simulink library "common_lib"  (R2021b)
settings: Solver=ode45  StartTime=0.0  StopTime=10.0  RelTol=1e-3
undefined symbols (not defined in the file or in its folder): ACCEL_PRE_MULT, C_C1GearNumbers, C_C1GearRatios, C_Calibration, C_DitherWaveform, C_GearOffset, C_GearRatioIn, C_GearRatioInverseOut, C_GearRatioOut, CLUTCH_INNER_LOOP_UPDATE_RATE, CONSTANT, DEGRADED_MODE_SIZE, Dem_EventStatusType, DiscIntNeverNeededParam, F_FAULT_ENUM, F_NOFAULT, F_OUTOFRANGE, F_RATELIMIT, FALSE, FMI14_SPECIAL_INSTRUCTIONS, FMI20_DATA_DRIFTED_HIGH, FMI21_DATA_DRIFTED_LOW, FMI29_RESERVED_FOR_SAE_ASSIGNMENT, FMI30_RESERVED_FOR_SAE_ASSIGNMENT, FMI31_CONDITION_EXISTS, FMI32_NO_FAULT, IC, k_accel, k_mean, LVDCU_OORH_FaultCntThd_C, MAX_UINT32, MEAN_PRE_MULT, NTriggers, QLTY_SIGNAL_FAILED, QLTY_SIGNAL_FULLY_FUNCTION, QLTY_SIGNAL_SUBSTITUTED_BY_1ST_CHOICE, QLTY_SIGNAL_SUBSTITUTED_BY_2ND_CHOICE, QLTY_SIGNAL_SUBSTITUTED_BY_3RD_CHOICE, QLTY_SIGNAL_SUBSTITUTED_BY_4TH_CHOICE, SAMPLE_TIME_100_mSec, SAMPLE_TIME_100_uSec, simin, T_TestPoint, TF_FALSE, TF_TRUE, TimeStep, TRUE, WORKSPACE_UPDATE_RATE, ZERO, Zero
libraries: $bdroot x120, simulink x27, simulink_extras x4, MBD_EPS_Local_Blockset x4
(part 5 of 10)

== system common_lib/Diagnostics/Calibration Enabled Debounce ==
  diagInput : Inport
  diagStartUpComp : Inport  Port=2
  diagMaxVal : Inport  Port=3
  diagMinVal : Inport  Port=4
  diagUpCnt : Inport  Port=5
  diagDnCnt : Inport  Port=6
  diagFaultCntThresh : Inport  Port=7
  diagPassCntThresh : Inport  Port=8
  diagDbncEnab : Inport  Port=9
  diagReset : Inport  Port=10
  diagEnable : Inport  Port=11
  diagHealEn : Inport  Port=12
  Calibration Enabled Debounce Boolean Input : $bdroot/Diagnostics/Calibration Enabled Debounce Boolean Input  SystemSampleTime=-1  VariantActivationTime=update diagram  Latency=0  AutoFrameSizeCalculation=off
  OR : Logic  Operator=OR  AllPortsSameDT=off  OutDataTypeStr=boolean
  Relational Operator : RelationalOperator  OutDataTypeStr=boolean  ZeroCross=off  RndMeth=Nearest
  Relational Operator1 : RelationalOperator  Operator=<=  OutDataTypeStr=boolean  ZeroCross=off  RndMeth=Nearest
  diagFaultStatus : Outport  OutputWhenDisabled=reset  InitialOutput=Dem_EventStatusType.DEM_EVENT_STATUS_INIT  VectorParamsAs1DForOutWhenUnconnected=off
  wires:
  diagHealEn/1 -> Calibration Enabled Debounce Boolean Input/10
  diagPassCntThresh/1 -> Calibration Enabled Debounce Boolean Input/7
  diagMaxVal/1 -> Relational Operator/2
  diagMinVal/1 -> Relational Operator1/2
  Relational Operator/1 -> OR/1
  Relational Operator1/1 -> OR/2
  diagInput/1 -> Relational Operator/1, Relational Operator1/1
  OR/1 -> Calibration Enabled Debounce Boolean Input/1
  diagStartUpComp/1 -> Calibration Enabled Debounce Boolean Input/2
  diagReset/1 -> Calibration Enabled Debounce Boolean Input/3
  diagEnable/1 -> Calibration Enabled Debounce Boolean Input/4
  diagDbncEnab/1 -> Calibration Enabled Debounce Boolean Input/5
  diagFaultCntThresh/1 -> Calibration Enabled Debounce Boolean Input/6
  diagUpCnt/1 -> Calibration Enabled Debounce Boolean Input/8
  diagDnCnt/1 -> Calibration Enabled Debounce Boolean Input/9
  Calibration Enabled Debounce Boolean Input/1 -> diagFaultStatus/1

== system common_lib/Diagnostics/Calibration Enabled Debounce Boolean Input ==
  diagInput : Inport
  diagStartUpComp : Inport  Port=2
  diagUpCnt : Inport  Port=3
  diagDnCnt : Inport  Port=4
  diagFaultCntThresh : Inport  Port=5
  diagPassCntThresh : Inport  Port=6
  diagDbncEnab : Inport  Port=7
  diagReset : Inport  Port=8
  diagEnable : Inport  Port=9
  diagHealEn : Inport  Port=10
  DiagFaultCounter : Subsystem
  diagFaultStatus : Outport  OutputWhenDisabled=reset  InitialOutput=Dem_EventStatusType.DEM_EVENT_STATUS_INIT  VectorParamsAs1DForOutWhenUnconnected=off
  diagFaultCnt : Outport  Port=2  OutputWhenDisabled=reset  InitialOutput=Dem_EventStatusType.DEM_EVENT_STATUS_INIT  VectorParamsAs1DForOutWhenUnconnected=off
  wires:
  DiagFaultCounter/1(diagFaultStatus) -> diagFaultStatus/1
  diagDnCnt/1 -> DiagFaultCounter/9(diagDnCnt)
  diagUpCnt/1 -> DiagFaultCounter/8(diagUpCnt)
  diagFaultCntThresh/1 -> DiagFaultCounter/6(diagFaultCntThresh)
  diagDbncEnab/1 -> DiagFaultCounter/5(diagDbncEnab)
  diagEnable/1 -> DiagFaultCounter/4(diagEnable)
  diagReset/1 -> DiagFaultCounter/3(diagReset)
  diagStartUpComp/1 -> DiagFaultCounter/2(diagStartUpComp)
  diagInput/1 -> DiagFaultCounter/1(diagFaultActive)
  diagPassCntThresh/1 -> DiagFaultCounter/7(diagPassCntThresh)
  diagHealEn/1 -> DiagFaultCounter/10(diagHealEn)
  DiagFaultCounter/2(diagFaultCnt) -> diagFaultCnt/1

== system common_lib/Diagnostics/Calibration Enabled MinMax OOR ==
  Input : Inport
  ULim : Inport  Port=2
  LLim : Inport  Port=3
  Cal_Enable : Inport  Port=4
  Ext_Fault : Inport  Port=5
  Enabled OOR : Subsystem  mask(Enabled OOR Subsystem){InitialValue=InitialValue, InDataType=single}
      mask prompts: InitialValue "Initial Value"; InDataType "Input Data Type"
      mask init:
      | DataType = get_param(gcb, 'InDataType');
      | Capture1 = [gcb '/OOR MinMax Capture/CL MinMax Capture'];
      | Capture2 = [gcb '/OOR MinMax Capture/CL MinMax Capture1'];
      | 
      | set_param(Capture1, 'InDataType', DataType);
      | set_param(Capture2, 'InDataType', DataType);
      mask TypeOptions InDataType: single | int16
  Switch : Switch  Threshold=0.5  ZeroCross=off
  Switch1 : Switch  Threshold=0.5  ZeroCross=off
  Out : Outport  VectorParamsAs1DForOutWhenUnconnected=off
  Max_Value : Outport  Port=2  VectorParamsAs1DForOutWhenUnconnected=off
  Min_Value : Outport  Port=3  VectorParamsAs1DForOutWhenUnconnected=off
  Fault : Outport  Port=4  VectorParamsAs1DForOutWhenUnconnected=off
  wires:
  Input/1 -> Enabled OOR/1(In), Switch/3
  ULim/1 -> Enabled OOR/2(ULim)
  LLim/1 -> Enabled OOR/3(LLim)
  Ext_Fault/1 -> Enabled OOR/4(Ext_Fault), Switch1/3
  Switch/1 -> Out/1
  Switch1/1 -> Fault/1
  Enabled OOR/1(Out) -> Switch/1
  Cal_Enable/1 -> Switch1/2, Switch/2, Enabled OOR/Enable
  Enabled OOR/2(Fault) -> Switch1/1
  Enabled OOR/3(Max) -> Max_Value/1
  Enabled OOR/4(Min) -> Min_Value/1

== system common_lib/Diagnostics/Calibration Enabled MinMax RLim ==
  Input : Inport
  Rate_Limit : Inport  Port=2
  Cal_Enable : Inport  Port=3
  Ext_Fault : Inport  Port=4
  Enabled RLim : Subsystem  mask(Enablede Rate Limit Fault Detection){IC=IC, TimeStep=TimeStep, InDataType=single}
      mask prompts: IC "Initial Condition"; TimeStep "Update Time"; InDataType "Input Data Type"
      mask init:
      | DataType = get_param(gcb, 'InDataType');
      | Capture1 = [gcb '/RLim MinMax Capture/CL MinMax Capture'];
      | Capture2 = [gcb '/RLim MinMax Capture/CL MinMax Capture1'];
      | 
      | set_param(Capture1, 'InDataType', DataType);
      | set_param(Capture2, 'InDataType', DataType);
      mask TypeOptions InDataType: single | int16
  Switch : Switch  Threshold=0.5  ZeroCross=off
  Switch1 : Switch  Threshold=0.5  ZeroCross=off
  Out : Outport  VectorParamsAs1DForOutWhenUnconnected=off
  Max Pos Rate : Outport  Port=2  VectorParamsAs1DForOutWhenUnconnected=off
  Max Neg Rate : Outport  Port=3  VectorParamsAs1DForOutWhenUnconnected=off
  Fault : Outport  Port=4  VectorParamsAs1DForOutWhenUnconnected=off
  wires:
  Cal_Enable/1 -> Switch/2, Switch1/2, Enabled RLim/Enable
  Input/1 -> Switch/3, Enabled RLim/1(In)
  Switch/1 -> Out/1
  Switch1/1 -> Fault/1
  Rate_Limit/1 -> Enabled RLim/2(RLim)
  Enabled RLim/1(out) -> Switch/1
  Enabled RLim/2(fault?) -> Switch1/1
  Ext_Fault/1 -> Enabled RLim/3(Ext_Fault), Switch1/3
  Enabled RLim/3(Max Pos Rate) -> Max Pos Rate/1
  Enabled RLim/4(Max Neg Rate) -> Max Neg Rate/1

== system common_lib/Diagnostics/Ccaller_DiagLv1 ==
  diagFaultActive : Inport
  diagStartUpComp : Inport  Port=2
  diagReset : Inport  Port=3
  diagEnable : Inport  Port=4
  diagDbncEnable : Inport  Port=5
  diagFaultCntThresh : Inport  Port=6
  diagPassCntThresh : Inport  Port=7
  diagUpCnt : Inport  Port=8
  diagDnCnt : Inport  Port=9
  diagHealEn : Inport  Port=10
  DiagDebounceLv1_CCaller : CCaller  FunctionName=DiagDebounceLv1  PortSpecificationStruct="%)30     .    <!<   8    (     @         %    \"     T    !     0         %  0 \"0    $    _    07)G3F%M90  4&]R=$YA;64 4V-O<&4     26YD97@     5'EP90      4VEZ90      27-';&]B86P   X   !     !@    @    $          4    (     0   !     !         !     0    9&EA9T9A=6QT0V]U;G1E<@X   !     !@    @    $          4    (     0   !     !         !     0    9&EA9T9A=6QT0V]U;G1E<@X   !     !@    @    $     ...(+7711 chars)"
  Unit Delay : UnitDelay  SampleTime=-1  HasFrameUpgradeWarning=on
      settings: AttributesFormatString=%<InitialCondition>
  Unit Delay1 : UnitDelay  InitialCondition=uint8(32)  SampleTime=-1  HasFrameUpgradeWarning=on
      settings: AttributesFormatString=%<InitialCondition>
  Unit Delay2 : UnitDelay  InitialCondition=false  SampleTime=-1  HasFrameUpgradeWarning=on
      settings: AttributesFormatString=%<InitialCondition>
  diagFaultStatus : Outport  VectorParamsAs1DForOutWhenUnconnected=off
  wires:
  diagUpCnt/1 -> DiagDebounceLv1_CCaller/11
  diagStartUpComp/1 -> DiagDebounceLv1_CCaller/5
  diagDnCnt/1 -> DiagDebounceLv1_CCaller/12
  diagReset/1 -> DiagDebounceLv1_CCaller/6
  diagFaultCntThresh/1 -> DiagDebounceLv1_CCaller/9
  diagFaultActive/1 -> DiagDebounceLv1_CCaller/4
  diagHealEn/1 -> DiagDebounceLv1_CCaller/13
  diagEnable/1 -> DiagDebounceLv1_CCaller/7
  diagDbncEnable/1 -> DiagDebounceLv1_CCaller/8
  diagPassCntThresh/1 -> DiagDebounceLv1_CCaller/10
  DiagDebounceLv1_CCaller/2 -> diagFaultStatus/1, Unit Delay1/1
  Unit Delay/1 -> DiagDebounceLv1_CCaller/1
  Unit Delay1/1 -> DiagDebounceLv1_CCaller/2
  DiagDebounceLv1_CCaller/3 -> Unit Delay2/1
  Unit Delay2/1 -> DiagDebounceLv1_CCaller/3
  DiagDebounceLv1_CCaller/1 -> Unit Delay/1

== system common_lib/Diagnostics/Ccaller_DiagLv2 ==
  diagFaultActive : Inport
  diagStartUpComp : Inport  Port=2
  diagReset : Inport  Port=3
  diagFaultCntThresh : Inport  Port=4
  diagUpCnt : Inport  Port=5
  diagDnCnt : Inport  Port=6
  diagHealEn : Inport  Port=7
  DiagDebounceLv2_CCaller : CCaller  FunctionName=DiagDebounceLv2  PortSpecificationStruct="%)30     .    8!$   8    (     @         %    \"     L    !     0         %  0 \"0    $    V    07)G3F%M90  4&]R=$YA;64 4V-O<&4     26YD97@     5'EP90      4VEZ90         .    ,     8    (    !          %    \"     $    #     0         0  , ;W5T  X    P    !@    @    $          4    (     0    ,    !         !   P!O=70 #@   #@    &    \"     0         !0    @    !    !@    $         $     8   !/=7 ...(+5614 chars)"
  Unit Delay : UnitDelay  InitialCondition=int16(0)  SampleTime=-1  HasFrameUpgradeWarning=on
      settings: AttributesFormatString=%<InitialCondition>
  Unit Delay1 : UnitDelay  InitialCondition=uint8(0)  SampleTime=-1  HasFrameUpgradeWarning=on
      settings: AttributesFormatString=%<InitialCondition>
  Unit Delay2 : UnitDelay  InitialCondition=int16(0)  SampleTime=-1  HasFrameUpgradeWarning=on
      settings: AttributesFormatString=%<InitialCondition>
  diagFaultStatus : Outport  VectorParamsAs1DForOutWhenUnconnected=off
  wires:
  Unit Delay2/1 -> DiagDebounceLv2_CCaller/3
  DiagDebounceLv2_CCaller/4 -> Unit Delay2/1
  Unit Delay1/1 -> DiagDebounceLv2_CCaller/2
  DiagDebounceLv2_CCaller/3 -> Unit Delay1/1
  Unit Delay/1 -> DiagDebounceLv2_CCaller/1
  DiagDebounceLv2_CCaller/2 -> Unit Delay/1
  diagHealEn/1 -> DiagDebounceLv2_CCaller/10
  diagFaultActive/1 -> DiagDebounceLv2_CCaller/4
  diagFaultCntThresh/1 -> DiagDebounceLv2_CCaller/7
  DiagDebounceLv2_CCaller/1 -> diagFaultStatus/1
  diagReset/1 -> DiagDebounceLv2_CCaller/6
  diagDnCnt/1 -> DiagDebounceLv2_CCaller/9
  diagStartUpComp/1 -> DiagDebounceLv2_CCaller/5
  diagUpCnt/1 -> DiagDebounceLv2_CCaller/8

== system common_lib/Diagnostics/DTNA_Diag ==
  diagInput : Inport
  diagStartUpComp : Inport  Port=2
  diagUpCnt : Inport  Port=3
  diagDnCnt : Inport  Port=4
  diagFaultCntThresh : Inport  Port=5
  diagPassCntThresh : Inport  Port=6
  diagDbncEnab : Inport  Port=7
  diagReset : Inport  Port=8
  diagEnable : Inport  Port=9
  diagHealEn : Inport  Port=10
  CC_Diag : Subsystem  VariantControl=CC_Diag
  S_Diag : Subsystem  AncestorBlock=common_lib/Diagnostics/Calibration Enabled Debounce Boolean Input  VariantControl=S_Diag
      settings: RTWSystemCode=Inline
  diagFaultStatus : Outport
  diagFaultCnt : Outport  Port=2

== system common_lib/Diagnostics/DiagFaultCounter ==
  diagFaultActive : Inport
  diagStartUpComp : Inport  Port=2
  diagReset : Inport  Port=3
  diagEnable : Inport  Port=4
  diagDbncEnab : Inport  Port=5
  diagFaultCntThresh : Inport  Port=6
  diagPassCntThresh : Inport  Port=7
  diagUpCnt : Inport  Port=8
  diagDnCnt : Inport  Port=9
  diagHealEn : Inport  Port=10
  DiagFaulCounter : Stateflow chart  TreatAsAtomicUnit=on
  diagFaultStatus : Outport  OutputWhenDisabled=reset  InitialOutput=Dem_EventStatusType.DEM_EVENT_STATUS_INIT  VectorParamsAs1DForOutWhenUnconnected=off
  wires:
  diagHealEn/1 -> DiagFaulCounter/10(diagHealEn)
  diagPassCntThresh/1 -> DiagFaulCounter/7(diagPassCntThresh)
  diagStartUpComp/1 -> DiagFaulCounter/2(diagStartUpComp)
  diagDbncEnab/1 -> DiagFaulCounter/5(diagDbncEnab)
  DiagFaulCounter/1(diagFaultStatus) -> diagFaultStatus/1
  diagEnable/1 -> DiagFaulCounter/4(diagEnable)
  diagDnCnt/1 -> DiagFaulCounter/9(diagDnCnt)
  diagUpCnt/1 -> DiagFaulCounter/8(diagUpCnt)
  diagReset/1 -> DiagFaulCounter/3(diagReset)
  diagFaultCntThresh/1 -> DiagFaulCounter/6(diagFaultCntThresh)
  diagFaultActive/1 -> DiagFaulCounter/1(diagFaultActive)

== system common_lib/Diagnostics/DiagcFltCumCnt ==
  diaginput : Inport
  diagStartUpComp : Inport  Port=2
  diagFaultCntThresh : Inport  Port=3
  diagReset : Inport  Port=4
  Add2 : Sum
  Constant{3,5,10..11} (4 alike) : Constant  Value=0
  Constant9 : Constant
  GreaterThanOrEqual2 : RelationalOperator  OutDataTypeStr=boolean  RndMeth=Simplest
  GreaterThanOrEqual3 : RelationalOperator  OutDataTypeStr=boolean  RndMeth=Simplest
  Increment Stored Integer1 : simulink/Additional Math & Discrete/Additional Math: Increment - Decrement/Increment Stored Integer
  Switch10 : Switch  Criteria=u2 ~= 0  Threshold=LVDCU_OORH_FaultCntThd_C  OutDataTypeStr=Inherit: Inherit via back propagation
  Switch11 : Switch  Criteria=u2 ~= 0  Threshold=LVDCU_OORH_FaultCntThd_C  OutDataTypeStr=Inherit: Inherit via back propagation
  Switch7 : Switch  Criteria=u2 ~= 0  Threshold=LVDCU_OORH_FaultCntThd_C +1
  Switch8 : Switch  Criteria=u2 > Threshold
  Switch9 : Switch  Criteria=u2 ~= 0  Threshold=1
  Unit Delay1 : UnitDelay  SampleTime=-1  HasFrameUpgradeWarning=on
  Unit Delay4 : UnitDelay  SampleTime=-1  HasFrameUpgradeWarning=on
  diagfaultStatus : Outport
  wires:
  Switch8/1 -> Switch9/3
  diaginput/1 -> Switch8/1
  diagStartUpComp/1 -> Switch8/3, Switch8/2
  Increment Stored Integer1/1 -> GreaterThanOrEqual2/2
  GreaterThanOrEqual2/1 -> Switch7/2
  Constant3/1 -> Switch7/1
  Constant5/1 -> Switch9/1
  Switch9/1 -> Add2/1
  Add2/1 -> GreaterThanOrEqual2/1, Switch7/3
  Unit Delay1/1 -> Add2/2
  Switch7/1 -> GreaterThanOrEqual3/1, Unit Delay1/1  "fault_count"
  diagFaultCntThresh/1 -> Increment Stored Integer1/1, GreaterThanOrEqual3/2
  GreaterThanOrEqual3/1 -> Switch10/2
  Constant9/1 -> Switch10/1
  Constant10/1 -> Switch10/3
  Switch11/1 -> Unit Delay4/1, diagfaultStatus/1
  diagReset/1 -> Switch11/2
  Switch10/1 -> Switch11/3
  Constant11/1 -> Switch11/1
  Unit Delay4/1 -> Switch9/2

== system common_lib/Diagnostics/DiagcFltCumUpCnt ==
  diaginput : Inport
  diagStartUpComp : Inport  Port=2
  diagUpCnt : Inport  Port=3
  diagFaultCntThresh : Inport  Port=4
  diagReset : Inport  Port=5
  Add2 : Sum
  Constant{3,5,10..11} (4 alike) : Constant  Value=0
  Constant9 : Constant
  Equal : RelationalOperator  Operator===  OutDataTypeStr=boolean  RndMeth=Simplest
  GreaterThanOrEqual2 : RelationalOperator  OutDataTypeStr=boolean  RndMeth=Simplest
  GreaterThanOrEqual3 : RelationalOperator  OutDataTypeStr=boolean  RndMeth=Simplest
  Increment Stored Integer1 : simulink/Additional Math & Discrete/Additional Math: Increment - Decrement/Increment Stored Integer
  Switch10 : Switch  Criteria=u2 ~= 0  Threshold=LVDCU_OORH_FaultCntThd_C  OutDataTypeStr=Inherit: Inherit via back propagation
  Switch11 : Switch  Criteria=u2 ~= 0  Threshold=LVDCU_OORH_FaultCntThd_C  OutDataTypeStr=Inherit: Inherit via back propagation
  Switch7 : Switch  Criteria=u2 ~= 0  Threshold=LVDCU_OORH_FaultCntThd_C +1
  Switch8 : Switch  Criteria=u2 > Threshold
  Switch9 : Switch  Criteria=u2 ~= 0  Threshold=1
  Unit Delay1 : UnitDelay  SampleTime=-1  HasFrameUpgradeWarning=on
  Unit Delay4 : UnitDelay  SampleTime=-1  HasFrameUpgradeWarning=on
  diagfaultStatus : Outport
  diagfaultCnt : Outport  Port=2
  wires:
  diagUpCnt/1 -> Equal/2
  Equal/1 -> Switch9/3
  Switch8/1 -> Equal/1
  diaginput/1 -> Switch8/1
  diagStartUpComp/1 -> Switch8/3, Switch8/2
  Increment Stored Integer1/1 -> GreaterThanOrEqual2/2
  GreaterThanOrEqual2/1 -> Switch7/2
  Constant3/1 -> Switch7/1
  Constant5/1 -> Switch9/1
  Switch9/1 -> Add2/1
  Add2/1 -> GreaterThanOrEqual2/1, Switch7/3
  Unit Delay1/1 -> Add2/2
  Switch7/1 -> diagfaultCnt/1, GreaterThanOrEqual3/1, Unit Delay1/1  "fault_count"
  diagFaultCntThresh/1 -> Increment Stored Integer1/1, GreaterThanOrEqual3/2
  GreaterThanOrEqual3/1 -> Switch10/2
  Constant9/1 -> Switch10/1
  Constant10/1 -> Switch10/3
  Switch11/1 -> Unit Delay4/1, diagfaultStatus/1
  diagReset/1 -> Switch11/2
  Switch10/1 -> Switch11/3
  Constant11/1 -> Switch11/1
  Unit Delay4/1 -> Switch9/2

== system common_lib/Diagnostics/DiagcFltResetCnt ==
  diaginput : Inport
  diagStartUpComp : Inport  Port=2
  diagFaultCntThresh : Inport  Port=3
  diagReset : Inport  Port=4
  Add2 : Sum
  Constant11 : Constant  Value=0
  Constant3 : Constant  Value=0
  Constant5 : Constant  Value=0
  Constant9 : Constant
  GreaterThanOrEqual2 : RelationalOperator  OutDataTypeStr=boolean  RndMeth=Simplest
  GreaterThanOrEqual3 : RelationalOperator  OutDataTypeStr=boolean  RndMeth=Simplest
  Increment Stored Integer1 : simulink/Additional Math & Discrete/Additional Math: Increment - Decrement/Increment Stored Integer
  Switch1 : Switch  Criteria=u2 > Threshold
  Switch10 : Switch  Criteria=u2 ~= 0  Threshold=LVDCU_OORH_FaultCntThd_C  OutDataTypeStr=Inherit: Inherit via back propagation
  Switch11 : Switch  Criteria=u2 ~= 0  Threshold=LVDCU_OORH_FaultCntThd_C  OutDataTypeStr=Inherit: Inherit via back propagation
  Switch7 : Switch  Criteria=u2 ~= 0  Threshold=LVDCU_OORH_FaultCntThd_C +1
  Switch8 : Switch  Criteria=u2 > Threshold
  Switch9 : Switch  Criteria=u2 ~= 0  Threshold=1
  Unit Delay1 : UnitDelay  SampleTime=-1  HasFrameUpgradeWarning=on
  Unit Delay2 : UnitDelay  SampleTime=-1  HasFrameUpgradeWarning=on
  Unit Delay4 : UnitDelay  SampleTime=-1  HasFrameUpgradeWarning=on
  diagfaultStatus : Outport
  wires:
  diaginput/1 -> Switch1/3, Switch1/2, Switch8/1
  diagStartUpComp/1 -> Switch8/3, Switch8/2
  Increment Stored Integer1/1 -> GreaterThanOrEqual2/2
  GreaterThanOrEqual2/1 -> Switch7/2
  Constant3/1 -> Switch7/1
  Constant5/1 -> Switch9/1
  Switch9/1 -> Add2/1
  Add2/1 -> GreaterThanOrEqual2/1, Switch7/3
  Switch7/1 -> GreaterThanOrEqual3/1, Unit Delay1/1  "LVDCU_OORH_fault_count"
  diagFaultCntThresh/1 -> Increment Stored Integer1/1, GreaterThanOrEqual3/2
  GreaterThanOrEqual3/1 -> Switch10/2
  Constant9/1 -> Switch10/1
  Switch11/1 -> Switch10/3
  Switch10/1 -> Unit Delay2/1, diagfaultStatus/1, Unit Delay4/1
  Unit Delay4/1 -> Switch9/2
  Unit Delay1/1 -> Switch1/1
  Switch1/1 -> Add2/2
  Switch8/1 -> Switch9/3
  Constant11/1 -> Switch11/1
  Unit Delay2/1 -> Switch11/3
  diagReset/1 -> Switch11/2

== system common_lib/Diagnostics/DiagcFltResetUpCnt ==
  diaginput : Inport
  diagStartUpComp : Inport  Port=2
  diagUpCnt : Inport  Port=3
  diagFaultCntThresh : Inport  Port=4
  diagReset : Inport  Port=5
  Add2 : Sum
  Constant11 : Constant  Value=0
  Constant3 : Constant  Value=0
  Constant5 : Constant  Value=0
  Constant9 : Constant
  Equal : RelationalOperator  Operator===  OutDataTypeStr=boolean  RndMeth=Simplest
  GreaterThanOrEqual2 : RelationalOperator  OutDataTypeStr=boolean  RndMeth=Simplest
  GreaterThanOrEqual3 : RelationalOperator  OutDataTypeStr=boolean  RndMeth=Simplest
  Increment Stored Integer1 : simulink/Additional Math & Discrete/Additional Math: Increment - Decrement/Increment Stored Integer
  Switch1 : Switch  Criteria=u2 > Threshold
  Switch10 : Switch  Criteria=u2 ~= 0  Threshold=LVDCU_OORH_FaultCntThd_C  OutDataTypeStr=Inherit: Inherit via back propagation
  Switch11 : Switch  Criteria=u2 ~= 0  Threshold=LVDCU_OORH_FaultCntThd_C  OutDataTypeStr=Inherit: Inherit via back propagation
  Switch7 : Switch  Criteria=u2 ~= 0  Threshold=LVDCU_OORH_FaultCntThd_C +1
  Switch8 : Switch  Criteria=u2 > Threshold
  Switch9 : Switch  Criteria=u2 ~= 0  Threshold=1
  Unit Delay1 : UnitDelay  SampleTime=-1  HasFrameUpgradeWarning=on
  Unit Delay2 : UnitDelay  SampleTime=-1  HasFrameUpgradeWarning=on
  Unit Delay4 : UnitDelay  SampleTime=-1  HasFrameUpgradeWarning=on
  diagfaultStatus : Outport
  wires:
  diaginput/1 -> Switch1/3, Switch1/2, Switch8/1
  diagStartUpComp/1 -> Switch8/3, Switch8/2
  Increment Stored Integer1/1 -> GreaterThanOrEqual2/2
  GreaterThanOrEqual2/1 -> Switch7/2
  Constant3/1 -> Switch7/1
  Constant5/1 -> Switch9/1
  Switch9/1 -> Add2/1
  Add2/1 -> GreaterThanOrEqual2/1, Switch7/3
  Switch7/1 -> GreaterThanOrEqual3/1, Unit Delay1/1  "LVDCU_OORH_fault_count"
  diagFaultCntThresh/1 -> Increment Stored Integer1/1, GreaterThanOrEqual3/2
  GreaterThanOrEqual3/1 -> Switch10/2
  Constant9/1 -> Switch10/1
  Switch11/1 -> Switch10/3
  Switch10/1 -> Unit Delay2/1, diagfaultStatus/1, Unit Delay4/1
  Unit Delay4/1 -> Switch9/2
  Unit Delay1/1 -> Switch1/1
  Switch1/1 -> Add2/2
  diagUpCnt/1 -> Equal/2
  Switch8/1 -> Equal/1
  Equal/1 -> Switch9/3
  Constant11/1 -> Switch11/1
  Unit Delay2/1 -> Switch11/3
  diagReset/1 -> Switch11/2

== system common_lib/Diagnostics/DiagcFltStSpaceHoldCnt ==
  diagFaultActive : Inport
  diagStartUpComp : Inport  Port=2
  diagUpCnt : Inport  Port=3
  diagFaultCntThresh : Inport  Port=4
  diagReset : Inport  Port=5
  diagcounter_hold : Stateflow chart  TreatAsAtomicUnit=on
  diagFaultStatus : Outport
  diagFaultCnt : Outport  Port=2
  wires:
  diagFaultActive/1 -> diagcounter_hold/1(diagFaultActive)
  diagcounter_hold/1(diagFaultStatus) -> diagFaultStatus/1
  diagFaultCntThresh/1 -> diagcounter_hold/4(diagFaultCntThresh)
  diagStartUpComp/1 -> diagcounter_hold/2(diagStartUpComp)
  diagcounter_hold/2(diagFaultCnt) -> diagFaultCnt/1
  diagUpCnt/1 -> diagcounter_hold/3(diagUpCnt)
  diagReset/1 -> diagcounter_hold/5(diagReset)

== system common_lib/Diagnostics/DiagcFltStSpaceRstCnt ==
  diagFaultActive : Inport
  diagStartUpComp : Inport  Port=2
  diagUpCnt : Inport  Port=3
  diagFaultCntThresh : Inport  Port=4
  diagReset : Inport  Port=5
  Chart : Stateflow chart  TreatAsAtomicUnit=on
  diagFaultStatus : Outport
  diagFaultCnt : Outport  Port=2
  wires:
  Chart/1(diagFaultStatus) -> diagFaultStatus/1
  diagFaultCntThresh/1 -> Chart/4(diagFaultCntThresh)
  diagReset/1 -> Chart/5(diagReset)
  diagStartUpComp/1 -> Chart/2(diagStartUpComp)
  diagFaultActive/1 -> Chart/1(diagFaultActive)
  diagUpCnt/1 -> Chart/3(diagUpCnt)
  Chart/2(diagFaultCnt) -> diagFaultCnt/1

== system common_lib/Diagnostics/ExtractValue ==
  in : Inport  OutDataTypeStr=Bus: BO_InputSignal
  Bus Selector : BusSelector  OutputSignals=value,FMI
  value : Outport  VectorParamsAs1DForOutWhenUnconnected=off
  FMI : Outport  Port=2  VectorParamsAs1DForOutWhenUnconnected=off
  wires:
  Bus Selector/2 -> FMI/1  "<FMI>"
  in/1 -> Bus Selector/1
  Bus Selector/1 -> value/1  "<value>"

== system common_lib/Diagnostics/FMIUpdate ==
  UpdateFaultStatus : Inport
  FMI_In : Inport  Port=2
  FMI_UpdateValue : Inport  Port=3
  Constant2 : Constant  Value=FMI32_NO_FAULT  SampleTime=-1
  Relational Operator3 : RelationalOperator  Operator=~=  ZeroCross=off  RndMeth=Nearest
  Switch : Switch  Threshold=0.5  ZeroCross=off
  Switch1 : Switch  Threshold=0.5  ZeroCross=off
  FMI_Out : Outport  VectorParamsAs1DForOutWhenUnconnected=off
  wires:
  Switch1/1 -> FMI_Out/1
  FMI_In/1 -> Switch/3, Switch1/1, Relational Operator3/1
  Relational Operator3/1 -> Switch1/2
  Switch/1 -> Switch1/3
  FMI_UpdateValue/1 -> Switch/1
  UpdateFaultStatus/1 -> Switch/2
  Constant2/1 -> Relational Operator3/2

== system common_lib/Diagnostics/FaultStatusUpdate ==
  FMI_In : Inport
  DriftLow : Inport  Port=2
  DriftHigh : Inport  Port=3
  SpecialInstructions : Inport  Port=4
  ConditionExists : Inport  Port=5
  DriftLowSubReqest : Inport  Port=6
  DriftLowSubReqest1 : Inport  Port=7
  Constant : Constant  Value=FMI14_SPECIAL_INSTRUCTIONS  SampleTime=-1
  Constant1 : Constant  Value=FMI21_DATA_DRIFTED_LOW  SampleTime=-1
  Constant2 : Constant  Value=FMI20_DATA_DRIFTED_HIGH  SampleTime=-1
  Constant3 : Constant  Value=FMI29_RESERVED_FOR_SAE_ASSIGNMENT  SampleTime=-1
  Constant4 : Constant  Value=FMI32_NO_FAULT  SampleTime=-1
  Constant5 : Constant  Value=FMI30_RESERVED_FOR_SAE_ASSIGNMENT  SampleTime=-1
  Constant6 : Constant  Value=FMI31_CONDITION_EXISTS  SampleTime=-1
  Relational Operator3 : RelationalOperator  Operator=~=  ZeroCross=off  RndMeth=Nearest
  Switch{,1..6} (7 alike) : Switch  Threshold=0.5  ZeroCross=off
  FMI_Out : Outport  VectorParamsAs1DForOutWhenUnconnected=off
  wires:
  Switch1/1 -> FMI_Out/1
  Constant4/1 -> Relational Operator3/2
  Switch/1 -> Switch1/3
  Relational Operator3/1 -> Switch1/2
  FMI_In/1 -> Relational Operator3/1, Switch1/1, Switch6/3
  Switch2/1 -> Switch/3
  Switch3/1 -> Switch2/3
  Switch4/1 -> Switch3/3
  DriftLow/1 -> Switch/2
  Constant1/1 -> Switch/1
  Constant2/1 -> Switch2/1
  DriftHigh/1 -> Switch2/2
  Constant/1 -> Switch3/1
  SpecialInstructions/1 -> Switch3/2
  Constant6/1 -> Switch4/1
  ConditionExists/1 -> Switch4/2
  Constant3/1 -> Switch5/1
  DriftLowSubReqest/1 -> Switch5/2
  Constant5/1 -> Switch6/1
  DriftLowSubReqest1/1 -> Switch6/2
  Switch6/1 -> Switch5/3
  Switch5/1 -> Switch4/3

== system common_lib/Diagnostics/KeepAlive ==
  State : Inport  OutDataTypeStr=boolean  PortDimensions=1
  A : Inport  Port=2  PortDimensions=1
  B : Inport  Port=3  PortDimensions=1
  Delay : UnitDelay  InitialCondition=false  SampleTime=-1  HasFrameUpgradeWarning=on
  Logical Operator : Logic  Operator=OR  AllPortsSameDT=off  OutDataTypeStr=boolean
  RelOp : RelationalOperator  Operator===  OutDataTypeStr=boolean  RndMeth=Nearest  InputSameDT=on
  Enable : Outport  OutDataTypeStr=boolean  PortDimensions=1  VectorParamsAs1DForOutWhenUnconnected=off
  Rel : Outport  Port=2  OutDataTypeStr=boolean  PortDimensions=1  VectorParamsAs1DForOutWhenUnconnected=off
  wires:
  RelOp/1 -> Logical Operator/2, Rel/1
  Logical Operator/1 -> Enable/1
  B/1 -> RelOp/2
  Delay/1 -> Logical Operator/1
  State/1 -> Delay/1
  A/1 -> RelOp/1

== system common_lib/Diagnostics/LogicBasedActivation ==
  note: Logic Based Activation
  Enable : Inport  OutDataTypeStr=boolean  PortDimensions=1
  DMToAdd : Inport  Port=2  OutDataTypeStr=uint32  PortDimensions=DM_SIZE
  Add : Inport  Port=3  OutDataTypeStr=boolean  PortDimensions=1
  DMPackedData_in : Inport  Port=4  OutDataTypeStr=uint32  PortDimensions=DM_SIZE
  Bitwise Operator : simulink/Logic and Bit Operations/Bitwise Operator  logicop=OR  UseBitMask=off  NumInputPorts=2  BitMask=bin2dec('11011001')  BitMaskRealWorld=Stored Integer
  Logical Operator1 : Logic  AllPortsSameDT=off
  Switch3 : Switch  Threshold=0.5  ZeroCross=off
  DMPackedData_out : Outport  OutDataTypeStr=uint32  PortDimensions=DM_SIZE  VectorParamsAs1DForOutWhenUnconnected=off
  wires:
  Switch3/1 -> DMPackedData_out/1
  Bitwise Operator/1 -> Switch3/1
  DMToAdd/1 -> Bitwise Operator/1
  DMPackedData_in/1 -> Bitwise Operator/2, Switch3/3
  Logical Operator1/1 -> Switch3/2
  Enable/1 -> Logical Operator1/1
  Add/1 -> Logical Operator1/2

== system common_lib/Diagnostics/LogicBasedDeactivation ==
  note: Logic Based Deactivation
  Enable : Inport  OutDataTypeStr=boolean  PortDimensions=1
  DMToRemove : Inport  Port=2  OutDataTypeStr=uint32  PortDimensions=DM_SIZE
  Remove : Inport  Port=3  OutDataTypeStr=boolean  PortDimensions=1
  DMPackedData_in : Inport  Port=4  OutDataTypeStr=uint32  PortDimensions=DM_SIZE
  Bitwise Operator : simulink/Logic and Bit Operations/Bitwise Operator  logicop=AND  UseBitMask=off  NumInputPorts=2  BitMask=bin2dec('11011001')  BitMaskRealWorld=Stored Integer
  Bitwise Operator1 : simulink/Logic and Bit Operations/Bitwise Operator  logicop=NOT  UseBitMask=off  BitMask=bin2dec('11011001')  BitMaskRealWorld=Stored Integer
  Logical Operator1 : Logic  AllPortsSameDT=off
  Switch3 : Switch  Threshold=0.5  ZeroCross=off
  DMPackedData_out : Outport  OutDataTypeStr=uint32  PortDimensions=DM_SIZE  VectorParamsAs1DForOutWhenUnconnected=off
  wires:
  Remove/1 -> Logical Operator1/2
  Enable/1 -> Logical Operator1/1
  Logical Operator1/1 -> Switch3/2
  DMPackedData_in/1 -> Switch3/3, Bitwise Operator/2
  DMToRemove/1 -> Bitwise Operator1/1
  Bitwise Operator/1 -> Switch3/1
  Switch3/1 -> DMPackedData_out/1
  Bitwise Operator1/1 -> Bitwise Operator/1

== system common_lib/Diagnostics/SetFMI ==
  FMI_in : Inport  OutDataTypeStr=uint8  PortDimensions=1
  Active1 : Inport  Port=2  OutDataTypeStr=boolean  PortDimensions=1
  Active2 : Inport  Port=3  OutDataTypeStr=boolean  PortDimensions=1
  Active3 : Inport  Port=4  OutDataTypeStr=boolean  PortDimensions=1
  Active4 : Inport  Port=5  OutDataTypeStr=boolean  PortDimensions=1
  Active5 : Inport  Port=6  OutDataTypeStr=boolean  PortDimensions=1
  Active6 : Inport  Port=7  OutDataTypeStr=boolean  PortDimensions=1
  Active7 : Inport  Port=8  OutDataTypeStr=boolean  PortDimensions=1
  Constant : Constant  Value=PRIORITY_1_FMI
  Constant1 : Constant  Value=PRIORITY_2_FMI
  Constant2 : Constant  Value=PRIORITY_3_FMI
  Constant3 : Constant  Value=PRIORITY_4_FMI
  Constant4 : Constant  Value=PRIORITY_5_FMI
  Constant5 : Constant  Value=PRIORITY_6_FMI
  Constant6 : Constant  Value=PRIORITY_7_FMI
  IF_ELSE_LADDER : Subsystem  TreatAsAtomicUnit=on
      settings: RTWSystemCode=Inline
  FMI_out : Outport  VectorParamsAs1DForOutWhenUnconnected=off
  wires:
  IF_ELSE_LADDER/1(FMI_out) -> FMI_out/1
  Active7/1 -> IF_ELSE_LADDER/8(Active7)
  Active6/1 -> IF_ELSE_LADDER/7(Active6)
  Active5/1 -> IF_ELSE_LADDER/6(Active5)
  Active4/1 -> IF_ELSE_LADDER/5(Active4)
  Active3/1 -> IF_ELSE_LADDER/4(Active3)
  Active2/1 -> IF_ELSE_LADDER/3(Active2)
  Active1/1 -> IF_ELSE_LADDER/2(Active1)
  FMI_in/1 -> IF_ELSE_LADDER/1(FMI_in)
  Constant6/1 -> IF_ELSE_LADDER/15(FMI_7)
  Constant5/1 -> IF_ELSE_LADDER/14(FMI_6)
  Constant4/1 -> IF_ELSE_LADDER/13(FMI_5)
  Constant3/1 -> IF_ELSE_LADDER/12(FMI_4)
  Constant2/1 -> IF_ELSE_LADDER/11(FMI_3)
  Constant1/1 -> IF_ELSE_LADDER/10(FMI_2)
  Constant/1 -> IF_ELSE_LADDER/9(FMI_1)

== system common_lib/Diagnostics/SignalSubstitution ==
  Signal_in : Inport  OutDataTypeStr=single  PortDimensions=1
  SignalFaulted : Inport  Port=2  OutDataTypeStr=boolean  PortDimensions=1
  FirstChoiceSubstitute : Inport  Port=3  OutDataTypeStr=single  PortDimensions=1
  FirstChoiceFaulted : Inport  Port=4  OutDataTypeStr=boolean  PortDimensions=1
  SecondChoiceSubstitute : Inport  Port=5  OutDataTypeStr=single  PortDimensions=1
  SecondChoiceFaulted : Inport  Port=6  OutDataTypeStr=boolean  PortDimensions=1
  ThirdChoiceSubstitute : Inport  Port=7  OutDataTypeStr=single  PortDimensions=1
  ThirdChoiceFaulted : Inport  Port=8  OutDataTypeStr=boolean  PortDimensions=1
  FourthChoiceSubstitute : Inport  Port=9  OutDataTypeStr=single  PortDimensions=1
  FourthChoiceFaulted : Inport  Port=10  OutDataTypeStr=boolean  PortDimensions=1
  FailedValue : Inport  Port=11  OutDataTypeStr=single  PortDimensions=1
  If : If  NumInputs=5  IfExpression=~u1  ElseIfExpressions=~u2, ~u3, ~u4, ~u5
  If Action Subsystem : Subsystem  TreatAsAtomicUnit=on
  If Action Subsystem1 : Subsystem  TreatAsAtomicUnit=on
  If Action Subsystem2 : Subsystem  TreatAsAtomicUnit=on
  If Action Subsystem3 : Subsystem  TreatAsAtomicUnit=on
  If Action Subsystem4 : Subsystem  TreatAsAtomicUnit=on
  If Action Subsystem5 : Subsystem  TreatAsAtomicUnit=on
  Merge : Merge  Inputs=6
  Merge1 : Merge  Inputs=6
  Signal_out : Outport  OutDataTypeStr=single  PortDimensions=1  VectorParamsAs1DForOutWhenUnconnected=off
  Qlty : Outport  Port=2  OutDataTypeStr=uint8  PortDimensions=1  VectorParamsAs1DForOutWhenUnconnected=off
  wires:
  If Action Subsystem2/2(Qlty) -> Merge1/3
  If Action Subsystem2/1(Signal) -> Merge/3
  If Action Subsystem1/2(Qlty) -> Merge1/2
  If Action Subsystem3/1(Signal) -> Merge/4
  Merge/1 -> Signal_out/1
  If Action Subsystem4/2(Qlty) -> Merge1/5
  If Action Subsystem/1(Signal) -> Merge/1
  If Action Subsystem4/1(Signal) -> Merge/5
  If Action Subsystem5/1(Signal) -> Merge/6
  If Action Subsystem1/1(Signal) -> Merge/2
  If Action Subsystem3/2(Qlty) -> Merge1/4
  If Action Subsystem/2(Qlty) -> Merge1/1
  If Action Subsystem5/2(Qlty) -> Merge1/6
  Merge1/1 -> Qlty/1
  If/3 -> If Action Subsystem2/Action
  Signal_in/1 -> If Action Subsystem/1(NoSubstitute)
  SecondChoiceSubstitute/1 -> If Action Subsystem2/1(SecondChoice)
  If/1 -> If Action Subsystem/Action
  FirstChoiceFaulted/1 -> If/2
  If/2 -> If Action Subsystem1/Action
  SecondChoiceFaulted/1 -> If/3
  FourthChoiceFaulted/1 -> If/5
  FirstChoiceSubstitute/1 -> If Action Subsystem1/1(FirstChoice)
  If/4 -> If Action Subsystem3/Action
  ThirdChoiceFaulted/1 -> If/4
  FailedValue/1 -> If Action Subsystem5/1(FailedValue)
  If/5 -> If Action Subsystem4/Action
  If/6 -> If Action Subsystem5/Action
  SignalFaulted/1 -> If/1
  FourthChoiceSubstitute/1 -> If Action Subsystem4/1(FourthChoice)
  ThirdChoiceSubstitute/1 -> If Action Subsystem3/1(ThirdChoice)
